simulink model "Assem"  (R2021b)
settings: Solver=VariableStepAuto  StartTime=0.0  StopTime=10.0  RelTol=1e-3
model workspace: external: MATLAB File C:\Users\Folk\Desktop\mbse\Test2\Assem_DataFile.m (data not in the file)
undefined symbols (not defined in the file): sigbuilder_block, smiData, X, Y, Z
libraries: sm_lib x31, nesl_utility x10, slpidlib x3
(part 2 of 2)

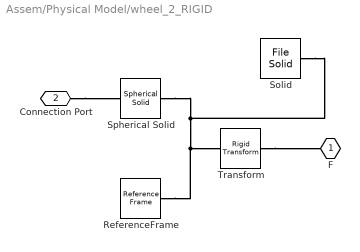
== system Assem/Physical Model/wheel_2_RIGID ==
  ReferenceFrame : sm_lib/Frames and Transforms/Reference Frame
  Solid : sm_lib/Body Elements/File Solid  ExtGeomFileName=wheel_Default_sldprt.STL  UnitType=Custom  ExtGeomFileUnits=mm  StepReaderType=HEX  ExportConvexHullGeometry=off  InertiaType=Custom  Mass=smiData.Solid(2).mass  MassUnits=kg  CenterOfMass=smiData.Solid(2).CoM  CenterOfMassUnits=mm  MomentsOfInertia=smiData.Solid(2).MoI  MomentsOfInertiaUnits=kg*mm^2  ProductsOfInertia=smiData.Solid(2).PoI  ProductsOfInertiaUnits=kg*mm^2  BasedOnType=DensityFromFile  Density=1000  DensityUnits=kg/m^3  DoExposeReferenceFrame=on  SerializedFrames=<Frames/>  GraphicType=FromGeometry  MarkerShape=Sphere  MarkerSize=10  GraphicVisPropType=SimpleVisualProperties  GraphicDiffuseColor=smiData.Solid(2).color  GraphicSpecularColor=[0.5 0.5 0.5 1.0]  GraphicAmbientColor=[0.15 0.15 0.15 1.0]  GraphicEmissiveColor=[0.0 0.0 0.0 1.0]  GraphicShininess=75  GraphicOpacity=smiData.Solid(2).opacity
  Spherical Solid : sm_lib/Body Elements/Spherical Solid  GraphicAmbientColor=[0.15 0.15 0.15 1.0]  BasedOnType=Density  CenterOfMass=[0 0 0]  CenterOfMassUnits=m  GraphicDiffuseColor=[0.5 0.5 0.5]  Density=1000  DensityUnits=kg/m^3  DoExposeReferenceFrame=on  GraphicEmissiveColor=[0.0 0.0 0.0 1.0]  ExportEntireGeometry=on  SerializedExposedGeometries=<ExposedGeometries><ExposedGeometry><RawGeometryId>entire</RawGeometryId><ExposedGeometryId>G</ExposedGeometryId></ExposedGeometry></ExposedGeometries>  SerializedFrames=<Frames/>  MarkerShape=Sphere  MarkerSize=10  GraphicType=None  InertiaType=CalculateFromGeometry  Mass=1  MassUnits=kg  MomentsOfInertia=[1 1 1]  MomentsOfInertiaUnits=kg*m^2  GraphicOpacity=1.0  ProductsOfInertia=[0 0 0]  ProductsOfInertiaUnits=kg*m^2  GraphicShininess=75  GraphicSpecularColor=[0.5 0.5 0.5 1.0]  SphereRadius=100  SphereRadiusUnits=mm  GraphicVisPropType=SimpleVisualProperties
  Transform : sm_lib/Frames and Transforms/Rigid Transform  TranslationMethod=Cartesian  TranslationStandardOffset=0  TranslationLengthUnit=mm  TranslationStandardAxis=+Z  TranslationCartesianOffset=smiData.RigidTransform(4).translation  TranslationROffset=0  TranslationROffsetUnits=m  TranslationZOffset=0  TranslationZOffsetUnits=m  TranslationThetaOffset=0  TranslationThetaOffsetUnits=deg  RotationMethod=ArbitraryAxis  RotationAngleUnits=rad  RotationStandardAxis=+Z  RotationAngle=smiData.RigidTransform(4).angle  RotationArbitraryAxis=smiData.RigidTransform(4).axis  FollAlignAxisA=+X  BaseAlignAxisA=+Y  FollAlignAxisB=+Y  BaseAlignAxisB=+Z  RotationSequenceAxes=FollowerAxes  RotationSequence=XYX  RotationSequenceAngles=[0 0 0]  RotationSequenceAnglesUnits=deg  RotationMatrix=[1 0 0; 0 1 0; 0 0 1]
  F : PMIOPort  Side=Left
  Connection Port : PMIOPort  Port=2  Side=Left
  connections:
  ReferenceFrame/RConn1 -- Solid/RConn1 -- Spherical Solid/RConn1 -- Transform/LConn1
  Transform/RConn1 -- F/RConn1
  Connection Port/RConn1 -- Spherical Solid/LConn1

== matlab function Assem/Kalman filter L/Kalman filter ==
  data: theta_k input; X1 output; X1 input; X2 input; P11 input; P12 input; P21 input; P22 input; X2 output; PP11 output; PP12 output; PP21 output; PP22 output; dP output
function [X1,X2,PP11,PP12,PP21,PP22,dP] = KalmanFilterFNC(theta_k,X1,X2,P11,P12,P21,P22)
%syms delta_t theta_k omega_k V_k Q x_k1 xp_hat_k x_hat_k P_hat_k yp_k R x11 x21 p11 p12 p21 p22 dt
dt = 0.0001;
omega_k = 0;
delta_t = dt;
A = [1 delta_t;0 1];
G = [delta_t*delta_t/2;delta_t];
C = [1 0];
Q = 6.800;
R = 0.01;
x_k = [theta_k;0]
%x_k = A*x_k1;
y_k = C*x_k;
x11 = X1;
x21 = X2;
x_hat_k = [x11;x21]
p11 = P11;
p12 = P12;
p21 = P21;
p22 = P22;
P_hat_k = [p11 p12;p21 p22];

%pred -------------------------------------

xp_hat_k = A*x_hat_k;
Pp_hat_k = A*P_hat_k*transpose(A) + G*Q*transpose(G);

%upadate

yp_k = C*xp_hat_k;
y_re_k = y_k - yp_k;
S_k = C*Pp_hat_k*transpose(C) + R;
K_k = Pp_hat_k*transpose(C)/(S_k);
x_hat_k1 = xp_hat_k+K_k*y_re_k;
P_hat_k1 = ([1 0;0 1]-(K_k*C))*Pp_hat_k;

%X1 = x_hat_k1(1);
%X2 = x_hat_k1(2);
%PP11 = P_hat_k1(1,1);
%PP12 = P_hat_k1(1,2);
%PP21 = P_hat_k1(2,1);
%PP22 =P_hat_k1(2,2);
X1 = X1 + X2*dt - ((X1 - theta_k + X2*dt)*(P11 + P21*dt + (Q*dt^4)/4 + dt*(P12 + P22*dt)))/(P11 + R + P21*dt + (Q*(dt^4))/4 + dt*(P12 + P22*dt));
	X2 = X2 - (((Q*(dt^3))/2 + P22*dt + P21)*(X1 - theta_k + X2*dt))/(P11 + R + P21*dt + (Q*(dt^4))/4 + dt*(P12 + P22*dt));
	PP11 = -((P11 + P21*dt + (Q*(dt^4))/4 + dt*(P12 + P22*dt))/(P11 + R + P21*dt + (Q*(dt^4))/4 + dt*(P12 + P22*dt)) - 1)*(P11 + P21*dt + (Q*(dt^4))/4 + dt*(P12 + P22*dt));
	PP12 = -((P11 + P21*dt + (Q*(dt^4))/4 + dt*(P12 + P22*dt))/(P11 + R + P21*dt + (Q*(dt^4))/4 + dt*(P12 + P22*dt)) - 1)*((Q*(dt^3))/2 + P22*dt + P12);
    PP21 = P21 + P22*dt + (Q*(dt^3))/2 - (((Q*(dt^3))/2 + P22*dt + P21)*(P11 + P21*dt + (Q*(dt^4))/4 + dt*(P12 + P22*dt)))/(P11 + R + P21*dt + (Q*(dt^4))/4 + dt*(P12 + P22*dt));
    PP22 = P22 + Q*(dt^2) - (((Q*(dt^3))/2 + P22*dt + P12)*((Q*(dt^3))/2 + P22*dt + P21))/(P11 + R + P21*dt + (Q*(dt^4))/4 + dt*(P12 + P22*dt));
    dP = det([PP11 PP12;PP21 PP22])

== matlab function Assem/IK ==
  data: v input; wL output; w input; R input; L input; wR output
function [wL,wR] = IK(v,w,R,L)
wL = (1/R)*(v-(w*L)/2);
wR = (1/R)*(v+(w*L)/2);

== matlab function Assem/Kalman filer R/Kalman filter ==
  data: theta_k input; X1 output; X1 input; X2 input; P11 input; P12 input; P21 input; P22 input; X2 output; PP11 output; PP12 output; PP21 output; PP22 output
function [X1,X2,PP11,PP12,PP21,PP22] = KalmanFilterFNC(theta_k,X1,X2,P11,P12,P21,P22)
%syms delta_t theta_k omega_k V_k Q x_k1 xp_hat_k x_hat_k P_hat_k yp_k R x11 x21 p11 p12 p21 p22 dt
dt =0.0001;
omega_k = 0;
delta_t = dt;
A = [1 delta_t;0 1];
G = [delta_t*delta_t/2;delta_t];
C = [1 0];
Q = 6.800;
R = 0.01;
x_k = [theta_k;0]
%x_k = A*x_k1;
y_k = C*x_k;
x11 = X1;
x21 = X2;
x_hat_k = [x11;x21]
p11 = P11;
p12 = P12;
p21 = P21;
p22 = P22;
P_hat_k = [p11 p12;p21 p22];

%pred -------------------------------------

xp_hat_k = A*x_hat_k;
Pp_hat_k = A*P_hat_k*transpose(A) + G*Q*transpose(G);

%upadate

yp_k = C*xp_hat_k;
y_re_k = y_k - yp_k;
S_k = C*Pp_hat_k*transpose(C) + R;
K_k = Pp_hat_k*transpose(C)/(S_k);
x_hat_k1 = xp_hat_k+K_k*y_re_k;
P_hat_k1 = ([1 0;0 1]-(K_k*C))*Pp_hat_k;

%X1 = x_hat_k1(1);
%X2 = x_hat_k1(2);
%PP11 = P_hat_k1(1,1);
%PP12 = P_hat_k1(1,2);
%PP21 = P_hat_k1(2,1);
%PP22 =P_hat_k1(2,2);
X1 = X1 + X2*dt - ((X1 - theta_k + X2*dt)*(P11 + P21*dt + (Q*dt^4)/4 + dt*(P12 + P22*dt)))/(P11 + R + P21*dt + (Q*(dt^4))/4 + dt*(P12 + P22*dt));
	X2 = X2 - (((Q*(dt^3))/2 + P22*dt + P21)*(X1 - theta_k + X2*dt))/(P11 + R + P21*dt + (Q*(dt^4))/4 + dt*(P12 + P22*dt));
	PP11 = -((P11 + P21*dt + (Q*(dt^4))/4 + dt*(P12 + P22*dt))/(P11 + R + P21*dt + (Q*(dt^4))/4 + dt*(P12 + P22*dt)) - 1)*(P11 + P21*dt + (Q*(dt^4))/4 + dt*(P12 + P22*dt));
	PP12 = -((P11 + P21*dt + (Q*(dt^4))/4 + dt*(P12 + P22*dt))/(P11 + R + P21*dt + (Q*(dt^4))/4 + dt*(P12 + P22*dt)) - 1)*((Q*(dt^3))/2 + P22*dt + P12);
    PP21 = P21 + P22*dt + (Q*(dt^3))/2 - (((Q*(dt^3))/2 + P22*dt + P21)*(P11 + P21*dt + (Q*(dt^4))/4 + dt*(P12 + P22*dt)))/(P11 + R + P21*dt + (Q*(dt^4))/4 + dt*(P12 + P22*dt));
    PP22 = P22 + Q*(dt^2) - (((Q*(dt^3))/2 + P22*dt + P12)*((Q*(dt^3))/2 + P22*dt + P21))/(P11 + R + P21*dt + (Q*(dt^4))/4 + dt*(P12 + P22*dt));

== matlab function Assem/MATLAB Function ==
  data: wL input; v output; wR input; R input; L input; w output
function [v,w] = FK(wL,wR,R,L)
v = (R/2)*(wL+wR);
w = (R/L)*(wR-wL);
